simulink model "Bluefin_Ver1"  (R2019b)
settings: Solver=ode4  StartTime=0.0  StopTime=200  FixedStep=0.1  RelTol=1e-3
libraries: simulink x1
settings Model: Creator=nguyenhd  LastModifiedBy=nguyenhd

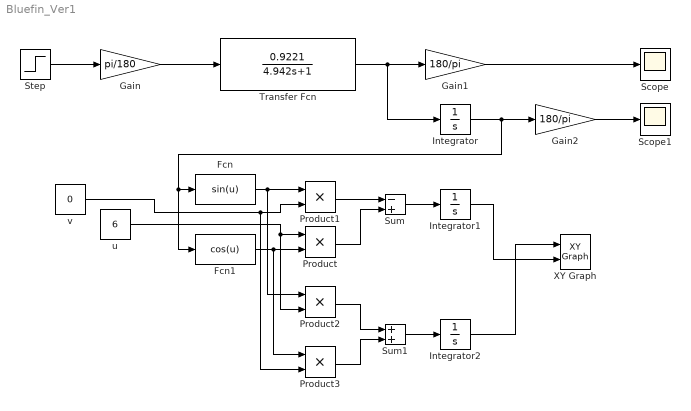
== system Bluefin_Ver1 ==
  Fcn : Fcn  Expr=sin(u)
  Fcn1 : Fcn  Expr=cos(u)
  Gain : Gain  Gain=pi/180
  Gain1 : Gain  Gain=180/pi
  Gain2 : Gain  Gain=180/pi
  Integrator : Integrator
  Integrator1 : Integrator
  Integrator2 : Integrator
  Product{,1..3} (4 alike) : Product
  Scope : Scope
  Scope1 : Scope
  Step : Step  Time=0  After=30  SampleTime=0
  Sum : Sum  Inputs=-+
  Sum1 : Sum
  Transfer Fcn : TransferFcn  Numerator=[0.9221]  Denominator=[4.942 1]
  XY Graph : simulink/Sinks/XY Graph  xmin=-100  xmax=100  ymin=-100  ymax=100  st=-1
  "u " : Constant  Value=6
  v : Constant  Value=0
  wires:
  Gain/1 -> Transfer Fcn/1
  Step/1 -> Gain/1
  Transfer Fcn/1 -> Integrator/1, Gain1/1
  Gain1/1 -> Scope/1
  Integrator/1 -> Fcn1/1, Fcn/1, Gain2/1
  Gain2/1 -> Scope1/1
  Fcn1/1 -> Product3/1, Product/2
  "u "/1 -> Product2/2, Product/1
  Fcn/1 -> Product2/1, Product1/1
  v/1 -> Product3/2, Product1/2
  Product1/1 -> Sum/1
  Product/1 -> Sum/2
  Product2/1 -> Sum1/1
  Product3/1 -> Sum1/2
  Sum/1 -> Integrator1/1
  Sum1/1 -> Integrator2/1
  Integrator2/1 -> XY Graph/1
  Integrator1/1 -> XY Graph/2
